simulink model "MPPTRegulator_Simulink"  (R2026a)
settings: Solver=VariableStepAuto
values from neighbouring files (symbols this model uses):
  a = 20    [MPPTRegulator.m]    (also in Ny_MPPTRegulator.m = 1)
  ad = 1/(n*Vt)    (= 0.5)    [MPPTRegulator.m]    (also in Ny_MPPTRegulator.m = 1.04166666667)
  b = 40    [MPPTRegulator.m]    (also in Ny_MPPTRegulator.m = 0.3)
  I_0 = 1e-2    (= 0.01)    [MPPTRegulator.m]    (also in Ny_MPPTRegulator.m = 0.0001)
  I_L = 5    [MPPTRegulator.m]    (also in Ny_MPPTRegulator.m)
  K_i = 5    [MPPTRegulator.m]    (also in Ny_MPPTRegulator.m = 2)
  K_P = 0.5    [MPPTRegulator.m]    (also in Ny_MPPTRegulator.m = 0.2)
  V_MMP = 9    [MPPTRegulator.m]    (also in Ny_MPPTRegulator.m = 8.24)
settings Model: Creator=tryma  LastModifiedBy=tryma

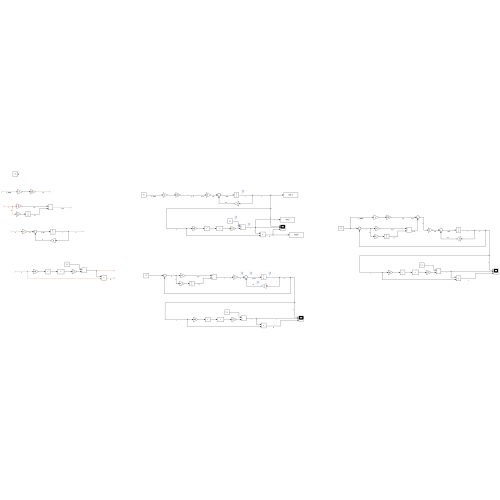
[thumbnail: Simulink's stored preview of the top-level diagram]
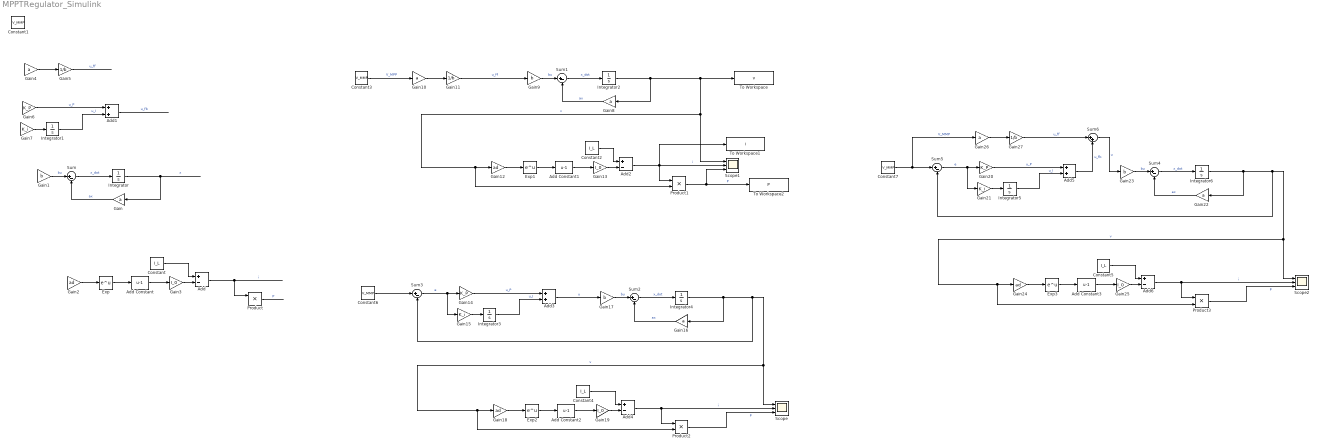
== system MPPTRegulator_Simulink ==
  Add{,2,4,6} (4 alike) : Sum  Inputs=+-
  Add Constant{,1..3} (4 alike) : Bias  Bias=-1  SaturateOnIntegerOverflow=off
  Add1 : Sum
  Add3 : Sum
  Add5 : Sum
  Constant{,2,4..5} (4 alike) : Constant  Value=I_L
  Constant{1,3,6..7} (4 alike) : Constant  Value=V_MMP
  Exp{,1..3} (4 alike) : Math
  Gain{,4,8,10,16,22,26} (7 alike) : Gain  Gain=a
  Gain{1,9,17,23} (4 alike) : Gain  Gain=b
  Gain11 : Gain  Gain=1/b
  Gain{2,12,18,24} (4 alike) : Gain  Gain=ad
  Gain{3,13,19,25} (4 alike) : Gain  Gain=I_0
  Gain14 : Gain  Gain=K_P
  Gain15 : Gain  Gain=K_i
  Gain20 : Gain  Gain=K_P
  Gain21 : Gain  Gain=K_i
  Gain27 : Gain  Gain=1/b
  Gain5 : Gain  Gain=1/b
  Gain6 : Gain  Gain=K_P
  Gain7 : Gain  Gain=K_i
  Integrator{,1..6} (7 alike) : Integrator
  Product{,1..3} (4 alike) : Product
  Scope : Scope  NumInputPorts=3
      settings: ActiveDisplayYMinimum=-4.6235559365827248  ActiveDisplayYMaximum=41.612003429244531
  Scope1 : Scope  NumInputPorts=3
      settings: ActiveDisplayYMinimum=-4.623557272869129  ActiveDisplayYMaximum=41.612015455822167
  Scope2 : Scope  NumInputPorts=3
      settings: ActiveDisplayYMinimum=-4.6236277312567093  ActiveDisplayYMaximum=41.612649581310393  DataLoggingVariableName=ScopeData2
  Sum{,1..5} (6 alike) : Sum  Inputs=|+-
  Sum6 : Sum  Inputs=|++
  To Workspace : ToWorkspace  VariableName=v  SaveFormat=Timeseries  SampleTime=-1
  To Workspace1 : ToWorkspace  VariableName=i  SaveFormat=Timeseries  SampleTime=-1
  To Workspace2 : ToWorkspace  VariableName=P  SaveFormat=Timeseries  SampleTime=-1
  wires:
  Sum/1 -> Integrator/1  "x_dot"
  Integrator/1 -> Gain/1  "x"
  Gain/1 -> Sum/2  "ax"
  Gain1/1 -> Sum/1  "bu"
  ? -> Gain1/1  "u"
  ? -> Product/2, Gain2/1  "x"
  Gain2/1 -> Exp/1
  Exp/1 -> Add Constant/1
  Add Constant/1 -> Gain3/1
  Constant/1 -> Add/1
  Gain3/1 -> Add/2
  Add/1 -> Product/1  "i"
  Product/1 -> ?  "P"
  Gain4/1 -> Gain5/1
  Gain5/1 -> ?  "u_ff"
  ? -> Gain4/1  "V_MMP"
  ? -> Gain7/1, Gain6/1  "e"
  Gain6/1 -> Add1/1  "u_P"
  Gain7/1 -> Integrator1/1
  Integrator1/1 -> Add1/2  "u_I"
  Add1/1 -> ?  "u_fb"
  Gain9/1 -> Sum1/1  "bu"
  Gain8/1 -> Sum1/2  "ax"
  Integrator2/1 -> To Workspace/1, Scope1/1, Product1/2, Gain12/1, Gain8/1  "v"
  Sum1/1 -> Integrator2/1  "x_dot"
  Constant3/1 -> Gain10/1  "V_MPP"
  Gain11/1 -> Gain9/1  "u_ff"
  Gain10/1 -> Gain11/1
  Product1/1 -> To Workspace2/1, Scope1/3  "P"
  Add2/1 -> Scope1/2, To Workspace1/1, Product1/1  "i"
  Gain13/1 -> Add2/2
  Add Constant1/1 -> Gain13/1
  Exp1/1 -> Add Constant1/1
  Gain12/1 -> Exp1/1
  Integrator3/1 -> Add3/2  "u_I"
  Gain15/1 -> Integrator3/1
  Gain14/1 -> Add3/1  "u_P"
  Sum3/1 -> Gain14/1, Gain15/1  "e"
  Add3/1 -> Gain17/1  "u"
  Gain17/1 -> Sum2/1  "bu"
  Gain16/1 -> Sum2/2  "ax"
  Integrator4/1 -> Gain16/1, Gain18/1, Product2/2, Scope/1, Sum3/2  "v"
  Sum2/1 -> Integrator4/1  "x_dot"
  Constant6/1 -> Sum3/1
  Product2/1 -> Scope/3  "P"
  Add4/1 -> Scope/2, Product2/1  "i"
  Gain19/1 -> Add4/2
  Constant4/1 -> Add4/1
  Add Constant2/1 -> Gain19/1
  Exp2/1 -> Add Constant2/1
  Gain18/1 -> Exp2/1
  Gain24/1 -> Exp3/1
  Exp3/1 -> Add Constant3/1
  Add Constant3/1 -> Gain25/1
  Constant5/1 -> Add6/1
  Gain25/1 -> Add6/2
  Add6/1 -> Product3/1, Scope2/2  "i"
  Product3/1 -> Scope2/3  "P"
  Sum4/1 -> Integrator6/1  "x_dot"
  Integrator6/1 -> Sum5/2, Scope2/1, Product3/2, Gain24/1, Gain22/1  "v"
  Gain22/1 -> Sum4/2  "ax"
  Gain23/1 -> Sum4/1  "bu"
  Sum5/1 -> Gain21/1, Gain20/1  "e"
  Gain20/1 -> Add5/1  "u_P"
  Gain21/1 -> Integrator5/1
  Integrator5/1 -> Add5/2  "u_I"
  Constant7/1 -> Gain26/1, Sum5/1  "V_MMP"
  Gain27/1 -> Sum6/1  "u_ff"
  Gain26/1 -> Gain27/1
  Add5/1 -> Sum6/2  "u_fb"
  Sum6/1 -> Gain23/1  "u"
  Constant2/1 -> Add2/1
